simulink model "RCAM_Simulink"  (R2023b)
settings: Solver=VariableStepAuto  StartTime=0.0  StopTime=TF  RelTol=1e-3
values from neighbouring files (symbols this model uses):
  RCAM = sim('RCAM_Simulink.slx')    [initialize.m]    (also in trimValidationRCAM.m)
  u1max = 25*pi/180    (= 0.436332312999)    [initialize.m]
  u1min = -25*pi/180    (= -0.436332312999)    [initialize.m]
  u2max = 10*pi/180    (= 0.174532925199)    [initialize.m]
  u2min = -25*pi/180    (= -0.436332312999)    [initialize.m]
  u3max = 30*pi/180    (= 0.523598775598)    [initialize.m]
  u3min = -30*pi/180    (= -0.523598775598)    [initialize.m]
  u4max = 10*pi/180    (= 0.174532925199)    [initialize.m]
  u4min = 0    [initialize.m]
  u5max = 10*pi/180    (= 0.174532925199)    [initialize.m]
  u5min = 0.5*pi/180    (= 0.00872664625997)    [initialize.m]
  UStar = ZStar(10:14)    [trimRCAM.m]    (also in trimValidationRCAM.m = temp.UStar; trim_values_straight_level.mat = [-1.04179321186e-09 -0.177950759919 -2.49290622986e-09 0.082)
  x0 = [85 ... (first row only)    [initialize.m]
settings Model: Creator=FlyingWing  LastModifiedBy=FlyingWing

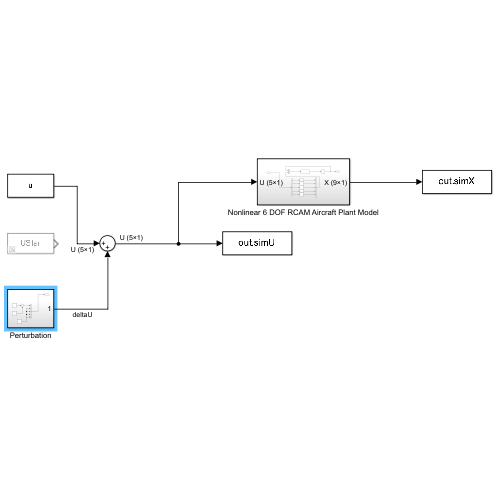
[thumbnail: Simulink's stored preview of the top-level diagram]
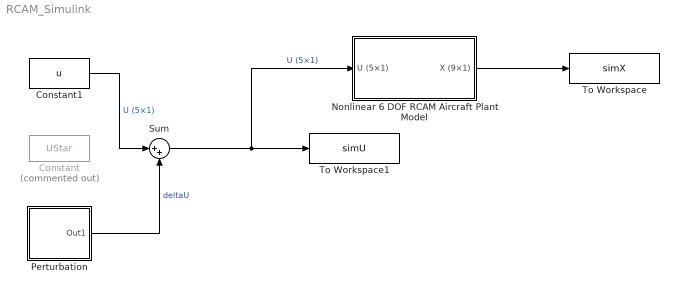
== system RCAM_Simulink ==
  Constant : Constant  Commented=on  Value=UStar
  Constant1 : Constant  Value=u
  Nonlinear 6 DOF RCAM Aircraft Plant Model : Subsystem
  Perturbation : Subsystem
  Sum : Sum  Inputs=|++
  To Workspace : ToWorkspace  VariableName=simX  SaveFormat=Timeseries  SampleTime=-1
  To Workspace1 : ToWorkspace  VariableName=simU  SaveFormat=Timeseries  SampleTime=-1
  wires:
  Sum/1 -> Nonlinear 6 DOF RCAM Aircraft Plant Model/1(U (5×1)), To Workspace1/1  "U (5×1)"
  Nonlinear 6 DOF RCAM Aircraft Plant Model/1(X (9×1)) -> To Workspace/1
  Constant1/1 -> Sum/1  "U (5×1)"
  Perturbation/1(Out1) -> Sum/2  "deltaU"

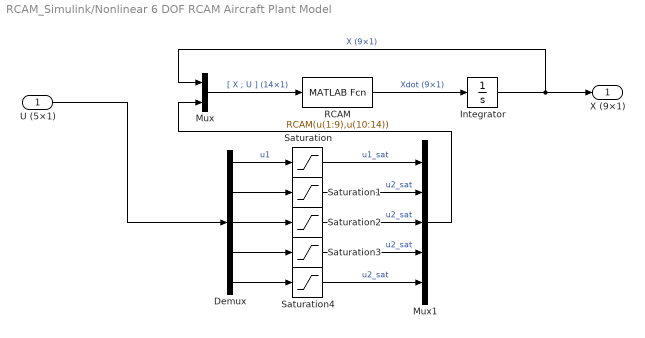
== system RCAM_Simulink/Nonlinear 6 DOF RCAM Aircraft Plant Model ==
  U (5×1) : Inport
  Demux : Demux  Outputs=5
  Integrator : Integrator  InitialCondition=x0
  Mux : Mux  Inputs=2
  Mux1 : Mux  Inputs=5
  RCAM : MATLABFcn  MATLABFcn=RCAM(u(1:9),u(10:14))
  Saturation : Saturate  UpperLimit=u1max  LowerLimit=u1min
  Saturation1 : Saturate  UpperLimit=u2max  LowerLimit=u2min
  Saturation2 : Saturate  UpperLimit=u3max  LowerLimit=u3min
  Saturation3 : Saturate  UpperLimit=u4max  LowerLimit=u4min
  Saturation4 : Saturate  UpperLimit=u5max  LowerLimit=u5min
  X (9×1) : Outport
  wires:
  Integrator/1 -> X (9×1)/1, Mux/1  "X (9×1)"
  Mux/1 -> RCAM/1  "[ X ; U ] (14×1)"
  RCAM/1 -> Integrator/1  "Xdot (9×1)"
  Saturation3/1 -> Mux1/4  "u2_sat"
  Saturation/1 -> Mux1/1  "u1_sat"
  Saturation4/1 -> Mux1/5  "u2_sat"
  Demux/1 -> Saturation/1  "u1"
  Demux/2 -> Saturation1/1
  Demux/4 -> Saturation3/1
  Demux/3 -> Saturation2/1
  U (5×1)/1 -> Demux/1
  Saturation2/1 -> Mux1/3  "u2_sat"
  Demux/5 -> Saturation4/1
  Mux1/1 -> Mux/2
  Saturation1/1 -> Mux1/2  "u2_sat"

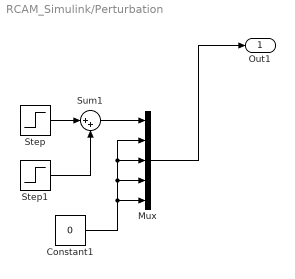
== system RCAM_Simulink/Perturbation ==
  Constant1 : Constant  Value=0
  Mux : Mux  Inputs=5
  Step : Step  Time=30  After=5*pi/180  SampleTime=0
  Step1 : Step  Time=30+1  After=-5*pi/180  SampleTime=0
  Sum1 : Sum  Inputs=|++
  Out1 : Outport
  wires:
  Constant1/1 -> Mux/5, Mux/4, Mux/2, Mux/3
  Step1/1 -> Sum1/2
  Step/1 -> Sum1/1
  Sum1/1 -> Mux/1
  Mux/1 -> Out1/1
